simulink model "NN_PD_2DOFRobot"  (R2024b)
settings: Solver=FixedStepAuto  StartTime=0.0  StopTime=40  FixedStep=0.01  RelTol=1e-3
libraries: fuzblock x2
settings Model: Creator=azonh  LastModifiedBy=ENVY

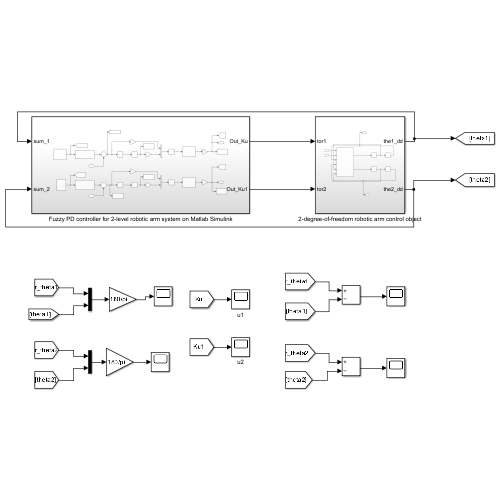
[thumbnail: Simulink's stored preview of the top-level diagram]
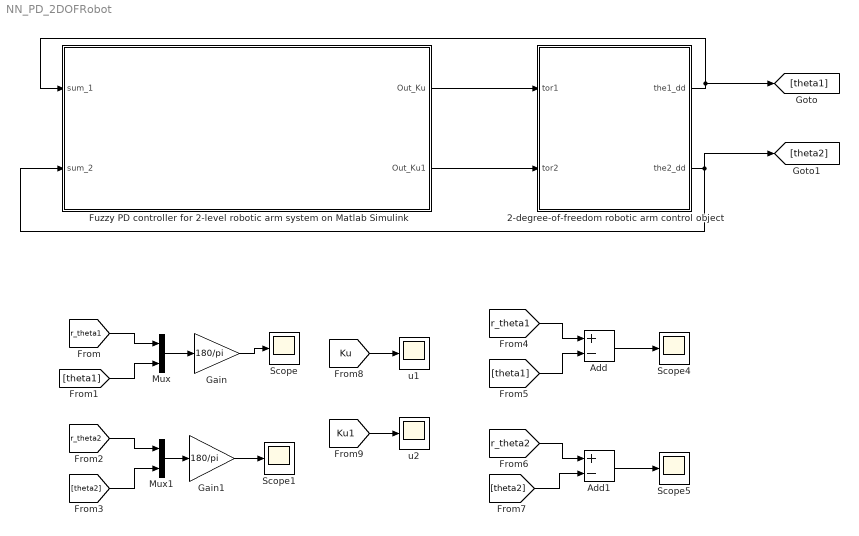
== system NN_PD_2DOFRobot ==
  2-degree-of-freedom robotic arm control object : Subsystem
  Add : Sum  Inputs=+-
  Add1 : Sum  Inputs=+-
  Fuzzy PD controller for 2-level robotic arm system on Matlab Simulink : Subsystem
  Gain : Gain  Gain=180/pi
  Gain1 : Gain  Gain=180/pi
  Mux : Mux  Inputs=2
  Mux1 : Mux  Inputs=2
  Scope{,1,4..5} (4 alike) : Scope
  u1 : Scope
  u2 : Scope
  wires:
  [r_theta2] -> Mux1/1
  Gain1/1 -> Scope1/1
  [theta2] -> Add1/2
  2-degree-of-freedom robotic arm control object/1(the1_dd) -> [theta1], Fuzzy PD controller for 2-level robotic arm system on Matlab Simulink/1(sum_1)
  [theta1] -> Mux/2
  Fuzzy PD controller for 2-level robotic arm system on Matlab Simulink/1(Out_Ku) -> 2-degree-of-freedom robotic arm control object/1(tor1)
  Gain/1 -> Scope/1
  [r_theta1] -> Mux/1
  [theta2] -> Mux1/2
  [r_theta1] -> Add/1
  Mux1/1 -> Gain1/1
  2-degree-of-freedom robotic arm control object/2(the2_dd) -> [theta2], Fuzzy PD controller for 2-level robotic arm system on Matlab Simulink/2(sum_2)
  [Ku1] -> u2/1
  Mux/1 -> Gain/1
  Fuzzy PD controller for 2-level robotic arm system on Matlab Simulink/2(Out_Ku1) -> 2-degree-of-freedom robotic arm control object/2(tor2)
  [theta1] -> Add/2
  [Ku] -> u1/1
  Add/1 -> Scope4/1
  [r_theta2] -> Add1/1
  Add1/1 -> Scope5/1

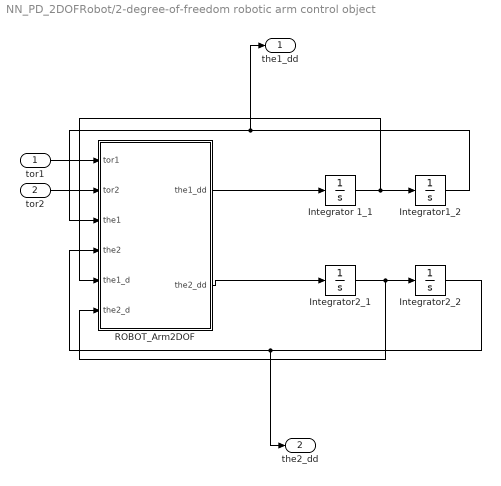
== system NN_PD_2DOFRobot/2-degree-of-freedom robotic arm control object ==
  tor1 : Inport
  tor2 : Inport  Port=2
  Integrator 1_1 : Integrator
  Integrator1_2 : Integrator
  Integrator2_1 : Integrator
  Integrator2_2 : Integrator
  ROBOT_Arm2DOF : MATLAB Function  TreatAsAtomicUnit=on
  the1_dd : Outport
  the2_dd : Outport  Port=2
  wires:
  Integrator1_2/1 -> the1_dd/1, ROBOT_Arm2DOF/3(the1)
  ROBOT_Arm2DOF/1(the1_dd) -> Integrator 1_1/1
  tor2/1 -> ROBOT_Arm2DOF/2(tor2)
  Integrator2_2/1 -> the2_dd/1, ROBOT_Arm2DOF/4(the2)
  Integrator2_1/1 -> ROBOT_Arm2DOF/6(the2_d), Integrator2_2/1
  tor1/1 -> ROBOT_Arm2DOF/1(tor1)
  Integrator 1_1/1 -> ROBOT_Arm2DOF/5(the1_d), Integrator1_2/1
  ROBOT_Arm2DOF/2(the2_dd) -> Integrator2_1/1

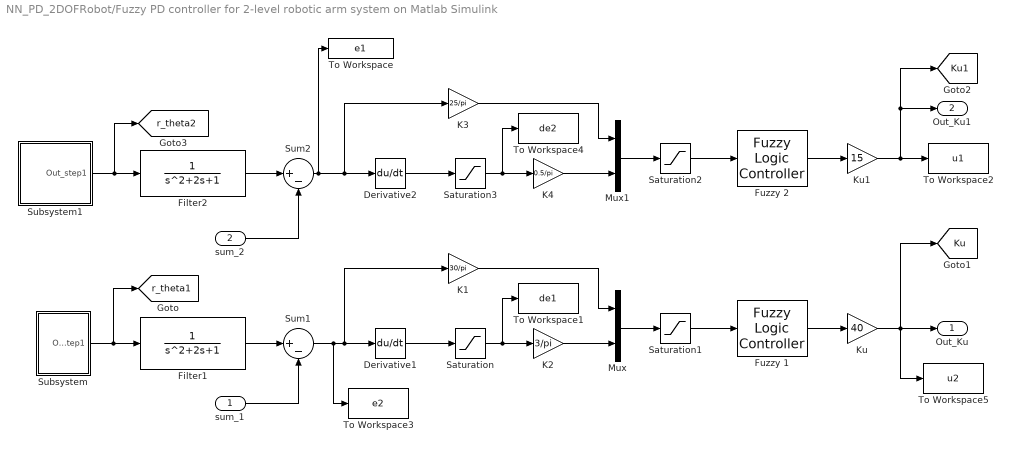
== system NN_PD_2DOFRobot/Fuzzy PD controller for 2-level robotic arm system on Matlab Simulink ==
  sum_1 : Inport
  sum_2 : Inport  Port=2
  Derivative1 : Derivative  CoefficientInTFapproximation=1
  Derivative2 : Derivative  CoefficientInTFapproximation=1
  Filter1 : TransferFcn
  Filter2 : TransferFcn
  Fuzzy 1 : fuzblock/Fuzzy Logic  Controller  FIS='FUZZY_ROBOT_ARM_3.fis'  OutputSampleNumber=101  DataType=double  FuzzifiedInputs=off  RuleFiringStrengths=off  RuleOutputs=off  AggregatedOutputs=off  SimulateUsing=Interpreted execution  OutOfRangeInputValueMessage=warning  NoRuleFiredMessage=warning  EmptyOutputFuzzySetMessage=warning
  Fuzzy 2 : fuzblock/Fuzzy Logic  Controller  FIS='FUZZY_ROBOT_ARM_3.fis'  OutputSampleNumber=101  DataType=double  FuzzifiedInputs=off  RuleFiringStrengths=off  RuleOutputs=off  AggregatedOutputs=off  SimulateUsing=Interpreted execution  OutOfRangeInputValueMessage=warning  NoRuleFiredMessage=warning  EmptyOutputFuzzySetMessage=warning
  K1 : Gain  Gain=30/pi
  K2 : Gain  Gain=3/pi
  K3 : Gain  Gain=25/pi
  K4 : Gain  Gain=0.5/pi
  Ku : Gain  Gain=40
  Ku1 : Gain  Gain=15
  Mux : Mux  Inputs=2
  Mux1 : Mux  Inputs=2
  Saturation{,1..3} (4 alike) : Saturate  UpperLimit=1  LowerLimit=-1
  Subsystem : Subsystem
  Subsystem1 : Subsystem
  Sum1 : Sum  Inputs=|+-
  Sum2 : Sum  Inputs=|+-
  To Workspace : ToWorkspace  VariableName=e1  SampleTime=-1
  To Workspace1 : ToWorkspace  VariableName=de1  SampleTime=-1
  To Workspace2 : ToWorkspace  VariableName=u1  SampleTime=-1
  To Workspace3 : ToWorkspace  VariableName=e2  SampleTime=-1
  To Workspace4 : ToWorkspace  VariableName=de2  SampleTime=-1
  To Workspace5 : ToWorkspace  VariableName=u2  SampleTime=-1
  Out_Ku : Outport
  Out_Ku1 : Outport  Port=2
  tag scope: Ku1=global, Ku=global, r_theta1=global, r_theta2=global
  wires:
  Filter1/1 -> Sum1/1
  Subsystem1/1(Out_step1) -> Filter2/1, [r_theta2]
  Filter2/1 -> Sum2/1
  Saturation1/1 -> Fuzzy 1/1
  Mux1/1 -> Saturation2/1
  Subsystem/1(Out_step1) -> [r_theta1], Filter1/1
  K1/1 -> Mux/1
  sum_2/1 -> Sum2/2
  sum_1/1 -> Sum1/2
  Sum2/1 -> To Workspace/1, K3/1, Derivative2/1
  Derivative1/1 -> Saturation/1
  Sum1/1 -> To Workspace3/1, K1/1, Derivative1/1
  Derivative2/1 -> Saturation3/1
  K3/1 -> Mux1/1
  Saturation3/1 -> To Workspace4/1, K4/1
  Saturation/1 -> To Workspace1/1, K2/1
  Mux/1 -> Saturation1/1
  K4/1 -> Mux1/2
  K2/1 -> Mux/2
  Saturation2/1 -> Fuzzy 2/1
  Fuzzy 2/1 -> Ku1/1
  Fuzzy 1/1 -> Ku/1
  Ku1/1 -> To Workspace2/1, [Ku1], Out_Ku1/1
  Ku/1 -> [Ku], Out_Ku/1, To Workspace5/1

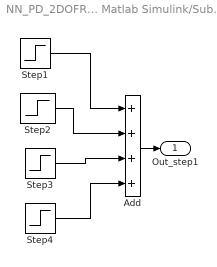
== system NN_PD_2DOFRobot/Fuzzy PD controller for 2-level robotic arm system on Matlab Simulink/Subsystem ==
  Add : Sum  Inputs=++++
  Step1 : Step  Time=0  After=-pi/4  SampleTime=0.01
  Step2 : Step  Time=10  After=pi/4  SampleTime=0.01
  Step3 : Step  Time=20  After=-pi/6  SampleTime=0.01
  Step4 : Step  Time=30  After=pi/3  SampleTime=0.01
  Out_step1 : Outport
  wires:
  Step4/1 -> Add/4
  Step2/1 -> Add/2
  Step1/1 -> Add/1
  Step3/1 -> Add/3
  Add/1 -> Out_step1/1

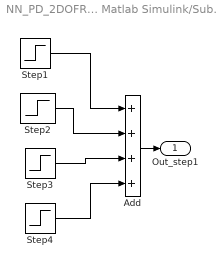
== system NN_PD_2DOFRobot/Fuzzy PD controller for 2-level robotic arm system on Matlab Simulink/Subsystem1 ==
  Add : Sum  Inputs=++++
  Step1 : Step  Time=0  After=pi/6  SampleTime=0.01
  Step2 : Step  Time=10  After=-pi/3  SampleTime=0.01  VectorParams1D=off
  Step3 : Step  Time=20  After=pi/6  SampleTime=0.01
  Step4 : Step  Time=30  After=-pi/4  SampleTime=0.01
  Out_step1 : Outport
  wires:
  Step4/1 -> Add/4
  Step2/1 -> Add/2
  Step1/1 -> Add/1
  Step3/1 -> Add/3
  Add/1 -> Out_step1/1

== matlab function NN_PD_2DOFRobot/2-degree-of-freedom robotic arm control object/ROBOT_Arm2DOF ==
  data: tor1 input; the1_dd output; tor2 input; the1 input; the2 input; the1_d input; the2_d input; the2_dd output
function [the1_dd, the2_dd] = fcn(tor1, tor2, the1, the2, the1_d, the2_d)
%#codegen
% Modèle dynamique du bras robotique 2-DoF
% Entrées: torques (Nm), positions (rad), vitesses (rad/s)
% Sorties: accélérations (rad/s²)

% --- Paramètres physiques ---
J1 = 0.05;      % Moment d'inertie joint 1 [kg·m²]
J2 = 0.05;      % Moment d'inertie joint 2 [kg·m²]
m1 = 1.0;       % Masse lien 1 [kg]
m2 = 1.0;       % Masse lien 2 [kg]
l1 = 1.0;       % Longueur lien 1 [m]
l2 = 1.0;       % Longueur lien 2 [m]
lc1 = 0.4;      % Distance CG lien 1 [m]
lc2 = 0.4;      % Distance CG lien 2 [m]
g = 9.81;       % Gravité [m/s²]

% --- Calculs intermédiaires ---
c2 = cos(the2);   % cos(theta2)
s2 = sin(the2);   % sin(theta2)
c12 = cos(the1 + the2);  % cos(theta1 + theta2)

% --- Matrice d'inertie M(theta) ---
% Élément M11
M11 = J1 + J2 + m1*lc1^2 + m2*(l1^2 + lc2^2 + 2*l1*lc2*c2);

% Élément M12 = M21
M12 = J2 + m2*(lc2^2 + l1*lc2*c2);

% Élément M22
M22 = J2 + m2*lc2^2;

% Construction de la matrice M
M = [M11, M12;
     M12, M22];  % Car M21 = M12 (matrice symétrique)

% --- Matrice de Coriolis/Centrifuge C(theta, theta_dot) ---
% Terme -m2*l1*lc2*s2
h = -m2*l1*lc2*s2;

% Construction de la matrice C
% Note: C est une matrice 2x2 selon la formule du manuel
C = [h*the2_d,     h*(the1_d + the2_d);
     -h*the1_d,    0];

% --- Vecteur de gravité G(theta) ---
G1 = (m1 + m2)*g*lc1*cos(the1) + m2*g*lc2*c12;
G2 = m2*g*lc2*c12;

G = [G1; G2];

% --- Vecteur d'état (vitesses) ---
theta_dot = [the1_d; the2_d];

% --- Calcul de l'accélération ---
% Équation: M * theta_ddot = tau - C * theta_dot - G
% Donc: theta_ddot = inv(M) * (tau - C*theta_dot - G)

tau = [tor1; tor2];  % Vecteur de couples

% Calcul du terme droit de l'équation
right_side = tau - C*theta_dot - G;

% Résolution pour theta_ddot (accélérations)
% Utilisation de l'opérateur backslash (plus stable que inv(M))
theta_ddot = M \ right_side;

% --- Extraction des sorties ---
the1_dd = theta_ddot(1);
the2_dd = theta_ddot(2);

end
